simulink model "GPCA_Extension"  (Simulink 7.9)
settings: Solver=ode45  StartTime=0.0  StopTime=inf  RelTol=1e-3
PreLoadFcn:
  | GPCA_Bus_Def
InitFcn:
  | script
values from neighbouring files (symbols this model uses):
  GOutputEvents = [0 0 0 0 0 0 0 0 0 0 0 0 0 0 0 0 0 0 0 0 0]    [script.m]
  GProgrammedDoseRate = 0    [script.m]
  GProgrammedVTBI = 0    [script.m]
libraries: simulink x6
(part 1 of 3)
settings Model: Creator=Yi Zhang  LastModifiedBy=paolo  BufferReuse=off
settings OptimizationCC: OptimizeBlockIOStorage=off  BufferReuse=off  ExpressionFolding=off  LocalBlockOutputs=off  InitFltsAndDblsToZero=on
settings DebuggingCC: FcnCallInpInsideContextMsg=Use local settings  UnconnectedInputMsg=none  UnconnectedOutputMsg=none  BusObjectLabelMismatch=none  StrictBusMsg=Warning
settings SFSimCC: SimParseCustomCode=off
settings GRTTargetCC: CombineOutputUpdateFcns=off  GRTInterface=on

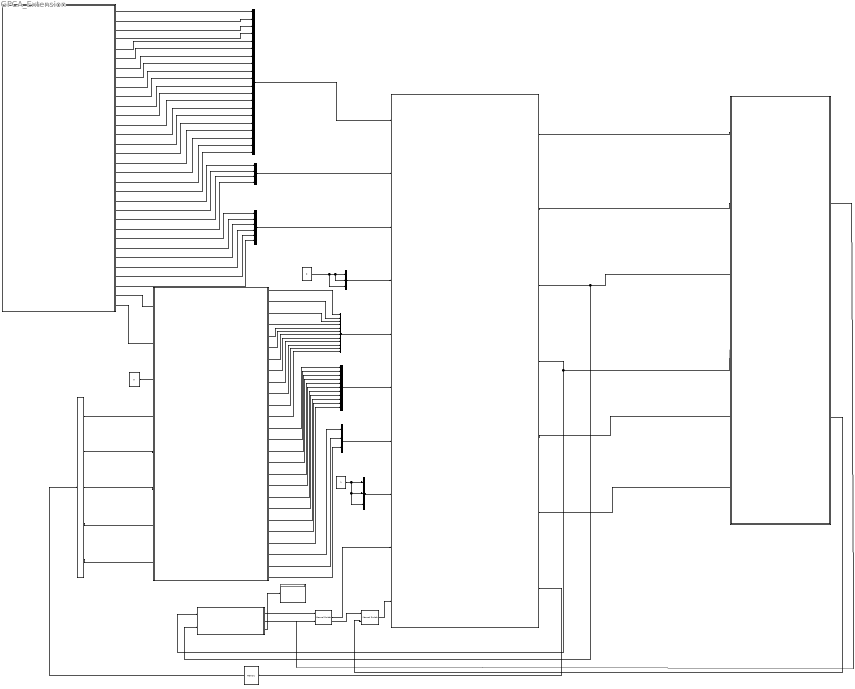
== system GPCA_Extension ==
  note: rrrvr
  1 : Constant  OutDataTypeStr=boolean
  2 : Constant  Value=0  OutDataTypeStr=boolean
  Bus Creator : BusCreator  Tag=DrugLIibraryInput  Description=Readings from the drug library  Inputs=20  OutDataTypeStr=Bus: DrugLibrary
      settings: AttributesFormatString=Drug Library Input
  Bus Creator1 : BusCreator  Description=Readings from the drug library  OutDataTypeStr=Bus: PatientInformation  NonVirtualBus=on
      settings: AttributesFormatString=Patient Information
  Bus Creator2 : BusCreator  Inputs=6  OutDataTypeStr=Bus: DrugInformation  NonVirtualBus=on
      settings: AttributesFormatString=Drug Information
  Bus Creator3 : BusCreator  Inputs=3  OutDataTypeStr=Bus: EnvironmentSensorSignals  NonVirtualBus=on
      settings: AttributesFormatString=Environment Sensor Signals
  Bus Creator4 : BusCreator  Inputs=12  OutDataTypeStr=Bus: HardwareSensorSignals  NonVirtualBus=on
      settings: AttributesFormatString=Hardware Sensor Signals
  Bus Creator5 : BusCreator  Inputs=11  OutDataTypeStr=Bus: InfusionSensorSignals  NonVirtualBus=on
      settings: AttributesFormatString=Infusion Sensor Signals
  Bus Creator7 : BusCreator  Inputs=3  OutDataTypeStr=Bus: InfusionStatus  NonVirtualBus=on
      settings: AttributesFormatString=Infusion Status
  Bus Creator8 : BusCreator  Inputs=3  OutDataTypeStr=Bus: PumpConfigurationsStatus  NonVirtualBus=on
      settings: AttributesFormatString=Pump Configuration Status
  Bus Selector : BusSelector  OutputSignals=signal1,signal3,signal2,O_ProgrammedFlowRate,O_ProgrammedVTBI
  Constant5 : Constant  Value=0
  Display GPCA-UI Port : Display
  Drug/Drug Library/Patient Information Reader : Subsystem
  GPCA Software Controller : Subsystem
  M2 : Memory  InheritSampleTime=on
  Manual Switch Infusion Parameters : simulink/Signal Routing/Manual Switch  sw=1  action=0  varsize=off
  Manual Switch User Actions : simulink/Signal Routing/Manual Switch  sw=1  action=0  varsize=off
  Pump Controller Subsystem : Subsystem
  UI : Subsystem
  WebSocketsBridge : Subsystem
  wires:
  Bus Creator/1 -> GPCA Software Controller/1(Drug Library Input)
  Bus Creator1/1 -> GPCA Software Controller/2(Patient Information Input)
  Bus Creator3/1 -> GPCA Software Controller/4(Environment Sensor Signals)
  Bus Creator4/1 -> GPCA Software Controller/5(Hardware Sensor Signals)
  Bus Creator7/1 -> GPCA Software Controller/7(Infusion Status Input)
  GPCA Software Controller/1(Drug Library Output) -> UI/1(Drug Lib)
  GPCA Software Controller/2(Patient Information Output) -> UI/2(Patient Info)
  GPCA Software Controller/4(Current State) -> WebSocketsBridge/1(CurrentState), UI/4(Current State)
  GPCA Software Controller/6(Alarming Condition) -> UI/6(Alarming Cond)
  GPCA Software Controller/3(Infusion Status Output) -> UI/3(Infusion Status), WebSocketsBridge/2(Infusion Status)
  GPCA Software Controller/5(Drug Information Output) -> UI/5(Drug Info)
  1/1 -> Bus Creator8/1, Bus Creator8/2, Bus Creator8/3
  Bus Creator8/1 -> GPCA Software Controller/8(Pump Configuration Status Input)
  Bus Creator5/1 -> GPCA Software Controller/6(Infusion Sensor Signals)
  GPCA Software Controller/7(Infusion Instructions Output) -> M2/1
  Bus Selector/3 -> Pump Controller Subsystem/6(Infusion Paused)  "<signal2>"
  Bus Selector/2 -> Pump Controller Subsystem/5(Bolus Requested)  "<signal3>"
  Bus Selector/5 -> Pump Controller Subsystem/8(Programmed VTBI)  "<O_ProgrammedVTBI>"
  Bus Selector/1 -> Pump Controller Subsystem/4(Infusion In Progress)  "<signal1>"
  Bus Selector/4 -> Pump Controller Subsystem/7(Programmed Flow Rate)  "<O_ProgrammedFlowRate>"
  Constant5/1 -> Pump Controller Subsystem/3(New Bag Inserted)
  Drug/Drug Library/Patient Information Reader/32(Bolus Time) -> Pump Controller Subsystem/2(Bolus Time)
  Drug/Drug Library/Patient Information Reader/31(Bolus Volume) -> Pump Controller Subsystem/1(Bolus Volume)
  Bus Creator2/1 -> GPCA Software Controller/3(Drug Information Input)
  Drug/Drug Library/Patient Information Reader/30(drugVolumeUnit) -> Bus Creator2/6
  Drug/Drug Library/Patient Information Reader/29(drugDoseUnit) -> Bus Creator2/5
  Drug/Drug Library/Patient Information Reader/28(drugConcentration) -> Bus Creator2/4
  Drug/Drug Library/Patient Information Reader/27(drugDiluentVolume) -> Bus Creator2/3
  Drug/Drug Library/Patient Information Reader/26(drugDoseAmount) -> Bus Creator2/2
  Drug/Drug Library/Patient Information Reader/25(drugName) -> Bus Creator2/1
  Drug/Drug Library/Patient Information Reader/24(patientWeight) -> Bus Creator1/4
  Drug/Drug Library/Patient Information Reader/23(patientGender) -> Bus Creator1/3
  Drug/Drug Library/Patient Information Reader/22(patientAge) -> Bus Creator1/2
  Drug/Drug Library/Patient Information Reader/21(patientName) -> Bus Creator1/1
  Drug/Drug Library/Patient Information Reader/20(drugConcentrationLowerSoftLimit) -> Bus Creator/20
  Drug/Drug Library/Patient Information Reader/19(drugConcentrationLowerHardLimit) -> Bus Creator/19
  Drug/Drug Library/Patient Information Reader/18(drugConcentrationUpperSoftLimit) -> Bus Creator/18
  Drug/Drug Library/Patient Information Reader/17(drugConcentrationUpperHardLimit) -> Bus Creator/17
  Drug/Drug Library/Patient Information Reader/16(drugConcentrationTypical) -> Bus Creator/16
  Drug/Drug Library/Patient Information Reader/15(vtbiUnit) -> Bus Creator/15
  Drug/Drug Library/Patient Information Reader/14(vtbiLowerSoftLimit) -> Bus Creator/14
  Drug/Drug Library/Patient Information Reader/1(drugID) -> Bus Creator/1
  Drug/Drug Library/Patient Information Reader/2(amount) -> Bus Creator/2
  Drug/Drug Library/Patient Information Reader/3(diluentVolume) -> Bus Creator/3
  Drug/Drug Library/Patient Information Reader/4(doseRateTypical) -> Bus Creator/4
  Drug/Drug Library/Patient Information Reader/5(doseRateUpperHardLimit) -> Bus Creator/5
  Drug/Drug Library/Patient Information Reader/6(doseRateUpperSoftLimit) -> Bus Creator/6
  Drug/Drug Library/Patient Information Reader/7(doseRateLowerHardLimit) -> Bus Creator/7
  Drug/Drug Library/Patient Information Reader/8(doseRateLowerSoftLimit) -> Bus Creator/8
  Drug/Drug Library/Patient Information Reader/9(doseRateUnit) -> Bus Creator/9
  Drug/Drug Library/Patient Information Reader/10(vtbiTypical) -> Bus Creator/10
  Drug/Drug Library/Patient Information Reader/11(vtbiUpperHardLimit) -> Bus Creator/11
  Drug/Drug Library/Patient Information Reader/12(vtbiUpperSoftLimit) -> Bus Creator/12
  Drug/Drug Library/Patient Information Reader/13(vtbiLowerHardLimit) -> Bus Creator/13
  2/1 -> Bus Creator3/1, Bus Creator3/2, Bus Creator3/3
  Pump Controller Subsystem/1(Log Failure) -> Bus Creator4/1
  Pump Controller Subsystem/2(Watchdog Interrupt) -> Bus Creator4/2
  Pump Controller Subsystem/3(Door Open) -> Bus Creator4/3
  Pump Controller Subsystem/4(Battery Depleted) -> Bus Creator4/4
  Pump Controller Subsystem/5(Battery Low) -> Bus Creator4/5
  Pump Controller Subsystem/6(Battery Charge Error) -> Bus Creator4/6
  Pump Controller Subsystem/7(VoltOutRange) -> Bus Creator4/7
  Pump Controller Subsystem/8(CPU Error) -> Bus Creator4/8
  Pump Controller Subsystem/9(RTCError) -> Bus Creator4/9
  Pump Controller Subsystem/10(MemoryCorrupted) -> Bus Creator4/10
  Pump Controller Subsystem/11(PumpTooHot) -> Bus Creator4/11
  Pump Controller Subsystem/12(PumpOverheat) -> Bus Creator4/12
  Pump Controller Subsystem/13(EmptyReservoir) -> Bus Creator5/1
  Pump Controller Subsystem/14(LowReservoir) -> Bus Creator5/2
  Pump Controller Subsystem/15(Occlusion) -> Bus Creator5/3
  Pump Controller Subsystem/16(RateTooHigh) -> Bus Creator5/4
  Pump Controller Subsystem/17(RateTooLow) -> Bus Creator5/5
  Pump Controller Subsystem/18(LessThanKVO) -> Bus Creator5/6
  Pump Controller Subsystem/19(RateVary) -> Bus Creator5/7
  Pump Controller Subsystem/20(Flow Rate Above Pump Capacity Alarm) -> Bus Creator5/8
  Pump Controller Subsystem/21(PauseLong) -> Bus Creator5/9
  Pump Controller Subsystem/22(PauseTooLong) -> Bus Creator5/10
  Pump Controller Subsystem/23(Air In Line) -> Bus Creator5/11
  Pump Controller Subsystem/24(Bolus In Progress) -> Bus Creator7/1
  Pump Controller Subsystem/25(TotalVolumeInfused) -> Bus Creator7/2
  Pump Controller Subsystem/26(Current Volume) -> Bus Creator7/3
  M2/1 -> Bus Selector/1
  WebSocketsBridge/1(User Actions) -> Manual Switch User Actions/1
  UI/1(User Actions) -> Manual Switch User Actions/2
  Manual Switch User Actions/1 -> GPCA Software Controller/9(User Actions)
  WebSocketsBridge/2(Infusion Parameters) -> Manual Switch Infusion Parameters/1
  Manual Switch Infusion Parameters/1 -> GPCA Software Controller/10(Infusion Parameters Input)
  UI/2(Infusion Parameters) -> Manual Switch Infusion Parameters/2
  WebSocketsBridge/3(Connection Port for the GPCA-UI) -> Display GPCA-UI Port/1

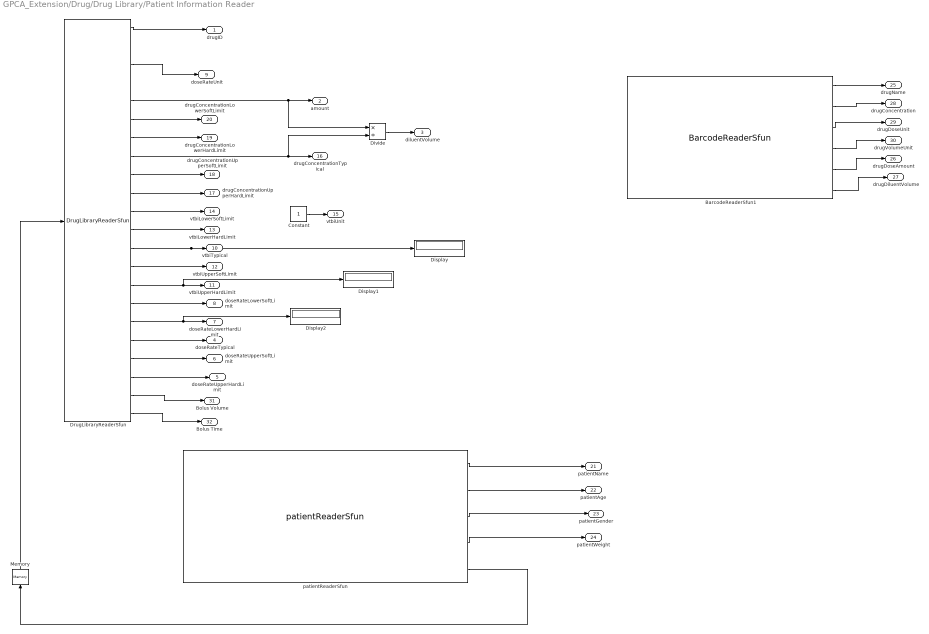
== system GPCA_Extension/Drug/Drug Library/Patient Information Reader ==
  BarcodeReaderSfun1 : S-Function  FunctionName=BarcodeReaderSfun  EnableBusSupport=off  mask(Legacy Function){SFunctionSpec=BarcodeReader(uint32 y1[1], double y2[1], uint32 y3[1], uint32 y4[1], double y5[1], double y6[1]), ShowSpec=on}
      mask prompts: ShowSpec "Display function specification"
      mask help:
      | This block allows you to call the legacy functions specified by the following Legacy Code Tool definition:
      | def.SFunctionName = 'BarcodeReaderSfun';
      | def.OutputFcnSpec = 'BarcodeReader(uint32 y1[1], double y2[1], uint32 y3[1], uint32 y4[1], double y5[1], double y6[1])';
      | def.StartFcnSpec = 'openFile()';
      | def.TerminateFcnSpec = 'closeFile()';
      | def.HeaderFiles = {'BarcodeReaderLCT.h'};
      | def.SourceFiles = {'BarcodeReaderLCT.c'};
      | def.SampleTime = 1;
      mask Help: <p>This block was generated automatically by the Legacy Code Tool. For detailed help on this tool, call<a href="matlab:legacy_code('help')"> legacy_code('help')</a>.</p>
      mask CallbackString:
      | |if strcmp(get_param(gcbh, 'ShowSpec'), 'on')
      |   set_param(gcbh, 'MaskDisplay', sprintf('fprintf(''%s'');', get_param(gcbh, 'SFunctionSpec')));
      | else
      |   set_param(gcbh, 'MaskDisplay', sprintf('fprintf(''%s'');', get_param(gcbh, 'FunctionName')));
      | end
      mask Display: fprintf('BarcodeReader(uint32 y1[1], double y2[1], uint32 y3[1], uint32 y4[1], double y5[1], double y6[1])');
  Constant : Constant  OutDataTypeStr=uint32
  Display : Display
  Display1 : Display
  Display2 : Display
  Divide : Product  Inputs=*/
  DrugLibraryReaderSfun : S-Function  FunctionName=DrugLibraryReaderSfun  EnableBusSupport=off  mask(Legacy Function){SFunctionSpec=DrugLibraryReader(uint32 u1[2], uint32 y1[1], uint32 y2[1], uint32 y3[1], uint32 y4[1], double  y5[1], double  y6[1], double  y7[1],double  y8[1],double  y9[1],double  y10[1],double  y11[1],double  y12[1], double  y13[1],double  y14[1],double  y15[1],double  y16[1],double  y17[1],double  y18[1],double  y19[1], double  y20[1],double  y21[1], uint32  y22[1]), ShowSpec=off}
      mask prompts: ShowSpec "Display function specification"
      mask help:
      | This block allows you to call the legacy functions specified by the following Legacy Code Tool definition:
      | def.SFunctionName = 'DrugLibraryReaderSfun';
      | def.OutputFcnSpec = 'DrugLibraryReader(uint32 u1[2], uint32 y1[1], uint32 y2[1], uint32 y3[1], uint32 y4[1], double  y5[1], double  y6[1], double  y7[1],double  y8[1],double  y9[1],double  y10[1],double  y11[1],double  y12[1], double  y13[1],double  y14[1],double  y15[1],double  y16[1],double  y17[1],double  y18[1],double  y19[1], double  y20[1],double  y21[1], uint32  y22[1])';
      | def.StartFcnSpec = 'openFile()';
      | def.TerminateFcnSpec = 'closeFile()';
      | def.HeaderFiles = {'DrugLibraryLCT.h'};
      | def.SourceFiles = {'DrugLibraryLCT.c'};
      | def.SampleTime = 1;
      mask Help: <p>This block was generated automatically by the Legacy Code Tool. For detailed help on this tool, call<a href="matlab:legacy_code('help')"> legacy_code('help')</a>.</p>
      mask CallbackString:
      | |if strcmp(get_param(gcbh, 'ShowSpec'), 'on')
      |   set_param(gcbh, 'MaskDisplay', sprintf('fprintf(''%s'');', get_param(gcbh, 'SFunctionSpec')));
      | else
      |   set_param(gcbh, 'MaskDisplay', sprintf('fprintf(''%s'');', get_param(gcbh, 'FunctionName')));
      | end
      mask Display: fprintf('DrugLibraryReaderSfun');
  Memory : Memory  InheritSampleTime=on
  patientReaderSfun : S-Function  FunctionName=patientReaderSfun  EnableBusSupport=off  mask(Legacy Function){SFunctionSpec=patientReader(uint32 y1[1], uint32 y2[1], uint32 y3[1], uint32 y4[1], uint32 y5[2]), ShowSpec=on}
      mask prompts: ShowSpec "Display function specification"
      mask help:
      | This block allows you to call the legacy functions specified by the following Legacy Code Tool definition:
      | def.SFunctionName = 'patientReaderSfun';
      | def.InitializeConditionsFcnSpec = 'randomizeSeed()';
      | def.OutputFcnSpec = 'patientReader(uint32 y1[1], uint32 y2[1], uint32 y3[1], uint32 y4[1], uint32 y5[2])';
      | def.StartFcnSpec = 'openFile()';
      | def.TerminateFcnSpec = 'closeFile()';
      | def.HeaderFiles = {'PatientDataReaderLCT.h'};
      | def.SourceFiles = {'PatientDataReaderLCT.c'};
      | def.SampleTime = 1;
      mask Help: <p>This block was generated automatically by the Legacy Code Tool. For detailed help on this tool, call<a href="matlab:legacy_code('help')"> legacy_code('help')</a>.</p>
      mask CallbackString:
      | |if strcmp(get_param(gcbh, 'ShowSpec'), 'on')
      |   set_param(gcbh, 'MaskDisplay', sprintf('fprintf(''%s'');', get_param(gcbh, 'SFunctionSpec')));
      | else
      |   set_param(gcbh, 'MaskDisplay', sprintf('fprintf(''%s'');', get_param(gcbh, 'FunctionName')));
      | end
      mask Display: fprintf('patientReader(uint32 y1[1], uint32 y2[1], uint32 y3[1], uint32 y4[1], uint32 y5[2])');
  drugID : Outport
  amount : Outport  Port=2
  diluentVolume : Outport  Port=3
  doseRateTypical : Outport  Port=4
  doseRateUpperHardLimit : Outport  Port=5
  doseRateUpperSoftLimit : Outport  Port=6
  doseRateLowerHardLimit : Outport  Port=7
  doseRateLowerSoftLimit : Outport  Port=8
  doseRateUnit : Outport  Port=9
  vtbiTypical : Outport  Port=10
  vtbiUpperHardLimit : Outport  Port=11
  vtbiUpperSoftLimit : Outport  Port=12
  vtbiLowerHardLimit : Outport  Port=13
  vtbiLowerSoftLimit : Outport  Port=14
  vtbiUnit : Outport  Port=15
  drugConcentrationTypical : Outport  Port=16
  drugConcentrationUpperHardLimit : Outport  Port=17
  drugConcentrationUpperSoftLimit : Outport  Port=18
  drugConcentrationLowerHardLimit : Outport  Port=19
  drugConcentrationLowerSoftLimit : Outport  Port=20
  patientName : Outport  Port=21
  patientAge : Outport  Port=22
  patientGender : Outport  Port=23
  patientWeight : Outport  Port=24
  drugName : Outport  Port=25
  drugDoseAmount : Outport  Port=26
  drugDiluentVolume : Outport  Port=27
  drugConcentration : Outport  Port=28
  drugDoseUnit : Outport  Port=29
  drugVolumeUnit : Outport  Port=30
  Bolus Volume : Outport  Port=31
  Bolus Time : Outport  Port=32
  wires:
  patientReaderSfun/5 -> Memory/1
  Memory/1 -> DrugLibraryReaderSfun/1
  Divide/1 -> diluentVolume/1
  Constant/1 -> vtbiUnit/1
  patientReaderSfun/1 -> patientName/1
  patientReaderSfun/2 -> patientAge/1
  patientReaderSfun/3 -> patientGender/1
  patientReaderSfun/4 -> patientWeight/1
  BarcodeReaderSfun1/1 -> drugName/1
  BarcodeReaderSfun1/2 -> drugConcentration/1
  BarcodeReaderSfun1/3 -> drugDoseUnit/1
  BarcodeReaderSfun1/4 -> drugVolumeUnit/1
  BarcodeReaderSfun1/5 -> drugDoseAmount/1
  BarcodeReaderSfun1/6 -> drugDiluentVolume/1
  DrugLibraryReaderSfun/1 -> drugID/1
  DrugLibraryReaderSfun/5 -> amount/1, Divide/1
  DrugLibraryReaderSfun/6 -> drugConcentrationLowerSoftLimit/1
  DrugLibraryReaderSfun/7 -> drugConcentrationLowerHardLimit/1
  DrugLibraryReaderSfun/8 -> drugConcentrationTypical/1, Divide/2
  DrugLibraryReaderSfun/9 -> drugConcentrationUpperSoftLimit/1
  DrugLibraryReaderSfun/10 -> drugConcentrationUpperHardLimit/1
  DrugLibraryReaderSfun/11 -> vtbiLowerSoftLimit/1
  DrugLibraryReaderSfun/12 -> vtbiLowerHardLimit/1
  DrugLibraryReaderSfun/13 -> vtbiTypical/1, Display/1
  DrugLibraryReaderSfun/14 -> vtbiUpperSoftLimit/1
  DrugLibraryReaderSfun/15 -> vtbiUpperHardLimit/1, Display1/1
  DrugLibraryReaderSfun/16 -> doseRateLowerSoftLimit/1
  DrugLibraryReaderSfun/17 -> doseRateLowerHardLimit/1, Display2/1
  DrugLibraryReaderSfun/18 -> doseRateTypical/1
  DrugLibraryReaderSfun/19 -> doseRateUpperSoftLimit/1
  DrugLibraryReaderSfun/20 -> doseRateUpperHardLimit/1
  DrugLibraryReaderSfun/3 -> doseRateUnit/1
  DrugLibraryReaderSfun/21 -> Bolus Volume/1
  DrugLibraryReaderSfun/22 -> Bolus Time/1

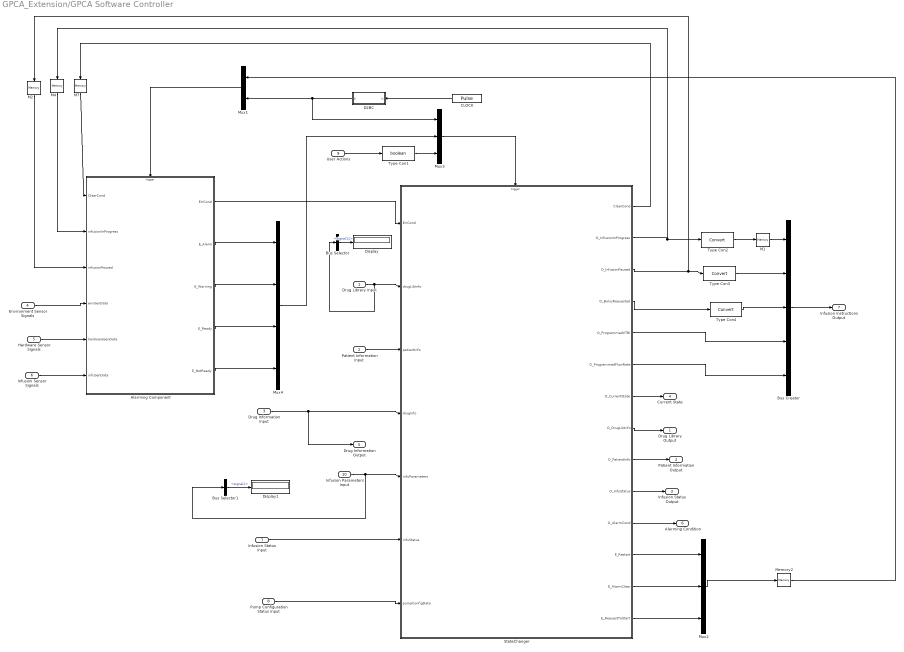
== system GPCA_Extension/GPCA Software Controller ==
  Drug Library Input : Inport
  Patient Information Input : Inport  Port=2
  Drug Information Input : Inport  Port=3
  Environment Sensor Signals : Inport  Port=4
  Hardware Sensor Signals : Inport  Port=5
  Infusion Sensor Signals : Inport  Port=6
  Infusion Status Input : Inport  Port=7
  Pump Configuration Status Input : Inport  Port=8
  User Actions : Inport  Port=9
  Infusion Parameters Input : Inport  Port=10
  Alarming Component : Stateflow chart  TreatAsAtomicUnit=on
  Bus Creator : BusCreator  Inputs=5  OutDataTypeStr=Bus: InfusionInstructions  NonVirtualBus=on
  Bus Selector : BusSelector  OutputSignals=signal11
  Bus Selector1 : BusSelector  OutputSignals=signal1
  CLOCK : DiscretePulseGenerator  PulseType=Time based  PulseWidth=50
  D2BC : MATLAB Function  TreatAsAtomicUnit=on
  Display : Display
  Display1 : Display
  M{1..2,4,7} (4 alike) : Memory  InheritSampleTime=on
  Memory2 : Memory  InheritSampleTime=on
  Mux1 : Mux  Inputs=2
  Mux2 : Mux  Inputs=3
  Mux3 : Mux  Inputs=3
  Mux4 : Mux
  StateChanger : Stateflow chart  TreatAsAtomicUnit=on
  Type Con1 : DataTypeConversion  OutDataTypeStr=boolean
  Type Con2 : DataTypeConversion
  Type Con3 : DataTypeConversion
  Type Con4 : DataTypeConversion
  Drug Library Output : Outport
  Patient Information Output : Outport  Port=2
  Infusion Status Output : Outport  Port=3
  Current State : Outport  Port=4
  Drug Information Output : Outport  Port=5
  Alarming Condition : Outport  Port=6
  Infusion Instructions Output : Outport  Port=7
  wires:
  StateChanger/1(ClearCond) -> M7/1
  Mux3/1 -> StateChanger/Trigger
  Mux1/1 -> Alarming Component/Trigger
  StateChanger/2(O_InfusionInProgress) -> M4/1, Type Con2/1
  Alarming Component/1(ErrCond) -> StateChanger/1(ErrCond)
  StateChanger/12(E_Restart) -> Mux2/1
  StateChanger/13(E_AlarmClear) -> Mux2/2
  StateChanger/14(E_RequestToStart) -> Mux2/3
  Mux2/1 -> Memory2/1
  CLOCK/1 -> D2BC/1(u)
  D2BC/1(y) -> Mux1/2, Mux3/1
  Alarming Component/2(E_Alarm) -> Mux4/1
  Alarming Component/3(E_Warning) -> Mux4/2
  Alarming Component/4(E_Ready) -> Mux4/3
  Alarming Component/5(E_NotReady) -> Mux4/4
  Mux4/1 -> Mux3/2
  Type Con2/1 -> M1/1
  Memory2/1 -> Mux1/1
  Environment Sensor Signals/1 -> Alarming Component/4(envSenData)
  Hardware Sensor Signals/1 -> Alarming Component/5(hardwareSenData)
  Infusion Sensor Signals/1 -> Alarming Component/6(infuSenData)
  Drug Library Input/1 -> StateChanger/2(drugLibInfo), Bus Selector/1
  Patient Information Input/1 -> StateChanger/3(patientInfo)
  Drug Information Input/1 -> StateChanger/4(drugInfo), Drug Information Output/1
  Infusion Parameters Input/1 -> StateChanger/5(infuParameters), Bus Selector1/1
  Infusion Status Input/1 -> StateChanger/6(infuStatus)
  Pump Configuration Status Input/1 -> StateChanger/7(pumpConfigData)
  StateChanger/11(O_AlarmCond) -> Alarming Condition/1
  StateChanger/7(O_CurrentState) -> Current State/1
  StateChanger/9(O_PatientInfo) -> Patient Information Output/1
  StateChanger/8(O_DrugLibInfo) -> Drug Library Output/1
  M1/1 -> Bus Creator/1
  StateChanger/3(O_InfusionPaused) -> M2/1, Type Con3/1
  Bus Creator/1 -> Infusion Instructions Output/1
  M7/1 -> Alarming Component/1(ClearCond)
  M4/1 -> Alarming Component/2(infusionInProgress)
  M2/1 -> Alarming Component/3(infusionPaused)
  StateChanger/4(O_BolusRequested) -> Type Con4/1
  StateChanger/5(O_ProgrammedVTBI) -> Bus Creator/4
  StateChanger/6(O_ProgrammedFlowRate) -> Bus Creator/5
  Type Con3/1 -> Bus Creator/2
  Type Con4/1 -> Bus Creator/3
  StateChanger/10(O_InfuStatus) -> Infusion Status Output/1
  Type Con1/1 -> Mux3/3
  User Actions/1 -> Type Con1/1
  Bus Selector/1 -> Display/1  "<signal11>"
  Bus Selector1/1 -> Display1/1  "<signal1>"

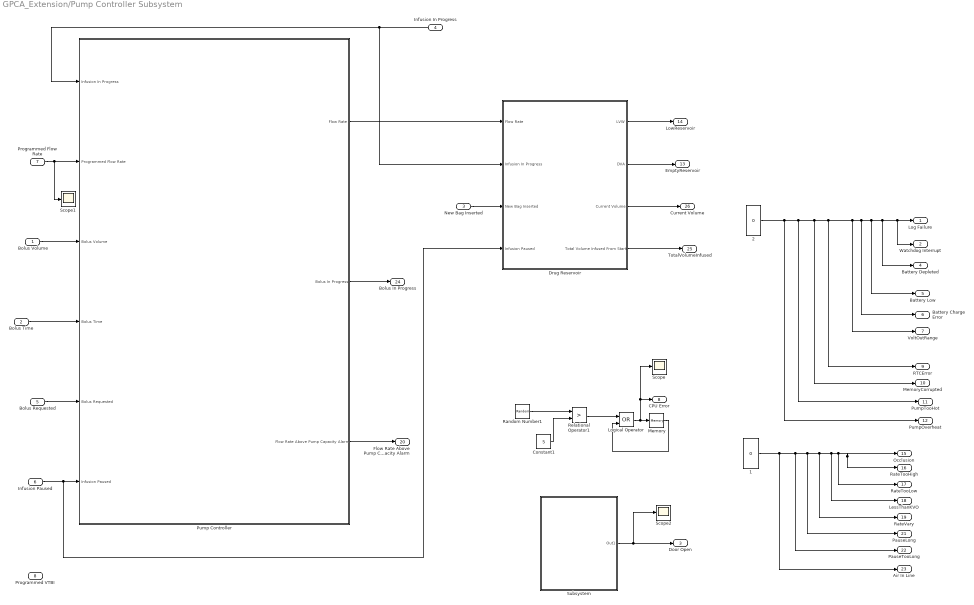
== system GPCA_Extension/Pump Controller Subsystem ==
  Bolus Volume : Inport
  Bolus Time : Inport  Port=2
  New Bag Inserted : Inport  Port=3
  Infusion In Progress : Inport  Port=4
  Bolus Requested : Inport  Port=5
  Infusion Paused : Inport  Port=6
  Programmed Flow Rate : Inport  Port=7
  Programmed VTBI : Inport  Port=8
  1 : Constant  Value=0  OutDataTypeStr=boolean
  2 : Constant  Value=0  OutDataTypeStr=boolean
  Constant1 : Constant  Value=5
  Drug Reservoir : Subsystem
  Logical Operator : Logic  Operator=OR  AllPortsSameDT=off  OutDataTypeStr=boolean
  Memory : Memory
  Pump Controller : Subsystem
  Random Number1 : RandomNumber  Mean=0.5
  Relational Operator1 : RelationalOperator  Operator=>  OutDataTypeStr=boolean
  Scope : Scope
      settings: YMin=1  YMax=1
  Scope1 : Scope
      settings: YMin=1.25  YMax=1.25
  Scope2 : Scope
      settings: YMin=-1  YMax=1  SaveName=ScopeData2
  Subsystem : Subsystem
  Log Failure : Outport
  Watchdog Interrupt : Outport  Port=2
  Door Open : Outport  Port=3
  Battery Depleted : Outport  Port=4
  Battery Low : Outport  Port=5
  Battery Charge Error : Outport  Port=6
  VoltOutRange : Outport  Port=7
  CPU Error : Outport  Port=8
  RTCError : Outport  Port=9
  MemoryCorrupted : Outport  Port=10
  PumpTooHot : Outport  Port=11
  PumpOverheat : Outport  Port=12
  EmptyReservoir : Outport  Port=13
  LowReservoir : Outport  Port=14
  Occlusion : Outport  Port=15
  RateTooHigh : Outport  Port=16
  RateTooLow : Outport  Port=17
  LessThanKVO : Outport  Port=18
  RateVary : Outport  Port=19
  Flow Rate Above Pump Capacity Alarm : Outport  Port=20
  PauseLong : Outport  Port=21
  PauseTooLong : Outport  Port=22
  Air In Line : Outport  Port=23
  Bolus In Progress : Outport  Port=24
  TotalVolumeInfused : Outport  Port=25
  Current Volume : Outport  Port=26
  wires:
  Bolus Requested/1 -> Pump Controller/5(Bolus Requested)
  Pump Controller/2(Bolus In Progress) -> Bolus In Progress/1
  Infusion Paused/1 -> Pump Controller/6(Infusion Paused), Drug Reservoir/4(Infusion Paused)
  New Bag Inserted/1 -> Drug Reservoir/3(New Bag Inserted)
  Drug Reservoir/3(Current Volume) -> Current Volume/1
  Drug Reservoir/2(DVA) -> EmptyReservoir/1
  Drug Reservoir/4(Total Volume Infused From Start) -> TotalVolumeInfused/1
  Infusion In Progress/1 -> Pump Controller/1(Infusion In Progress), Drug Reservoir/2(Infusion In Progress)
  Programmed Flow Rate/1 -> Pump Controller/2(Programmed Flow Rate), Scope1/1
  Drug Reservoir/1(LVW) -> LowReservoir/1
  Pump Controller/3(Flow Rate Above Pump Capacity Alarm) -> Flow Rate Above Pump Capacity Alarm/1
  Bolus Time/1 -> Pump Controller/4(Bolus Time)
  Bolus Volume/1 -> Pump Controller/3(Bolus Volume)
  2/1 -> RTCError/1, Battery Charge Error/1, Battery Low/1, Log Failure/1, Watchdog Interrupt/1, Battery Depleted/1, VoltOutRange/1, MemoryCorrupted/1, PumpTooHot/1, PumpOverheat/1
  1/1 -> RateTooLow/1, RateTooHigh/1, Occlusion/1, LessThanKVO/1, RateVary/1, PauseLong/1, PauseTooLong/1, Air In Line/1
  Pump Controller/1(Flow Rate) -> Drug Reservoir/1(Flow Rate)
  Random Number1/1 -> Relational Operator1/1
  Constant1/1 -> Relational Operator1/2
  Relational Operator1/1 -> Logical Operator/1
  Logical Operator/1 -> Memory/1, CPU Error/1, Scope/1
  Memory/1 -> Logical Operator/2
  Subsystem/1(Out1) -> Scope2/1, Door Open/1

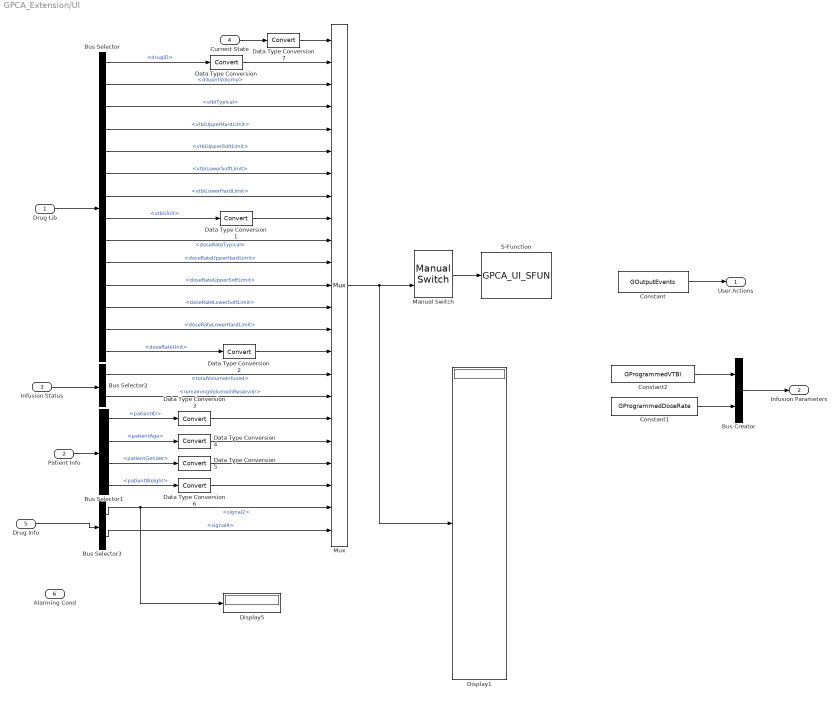
== system GPCA_Extension/UI ==
  Drug Lib : Inport
  Patient Info : Inport  Port=2
  Infusion Status : Inport  Port=3
  Current State : Inport  Port=4
  Drug Info : Inport  Port=5
  Alarming Cond : Inport  Port=6
  Bus Creator : BusCreator  Inputs=2  OutDataTypeStr=Bus: InfusionParameters
  Bus Selector : BusSelector  OutputSignals=drugID,diluentVolume,vtbiTypical,vtbiUpperHardLimit,vtbiUpperSoftLimit,vtbiLowerSoftLimit,vtbiLowerHardLimit,vtbiUnit,doseRateTypical,doseRateUpperHardLimit,doseRateUpperSoftLimit,doseRateLowerSoftLimit,doseRateLowerHardLimit,doseRateUnit
  Bus Selector1 : BusSelector  OutputSignals=patientID,patientAge,patientGender,patientWeight
  Bus Selector2 : BusSelector  OutputSignals=totalVolumeInfused,remainingVolumeInReservoir
  Bus Selector3 : BusSelector  OutputSignals=signal2,signal4
  Constant : Constant  Value=GOutputEvents
  Constant1 : Constant  Value=GProgrammedDoseRate
  Constant2 : Constant  Value=GProgrammedVTBI
  Data Type Conversion{,1..7} (8 alike) : DataTypeConversion
  Display1 : Display
  Display5 : Display
  Manual Switch : simulink/Signal Routing/Manual Switch  sw=0  action=0  varsize=off
  Mux : Mux  Inputs=23
  S-Function : S-Function  FunctionName=GPCA_UI_SFUN  EnableBusSupport=off
  User Actions : Outport
  Infusion Parameters : Outport  Port=2
  wires:
  Current State/1 -> Data Type Conversion7/1
  Drug Lib/1 -> Bus Selector/1
  Bus Selector/1 -> Data Type Conversion/1  "<drugID>"
  Bus Selector/2 -> Mux/3  "<diluentVolume>"
  Bus Selector/3 -> Mux/4  "<vtbiTypical>"
  Bus Selector/4 -> Mux/5  "<vtbiUpperHardLimit>"
  Bus Selector/5 -> Mux/6  "<vtbiUpperSoftLimit>"
  Bus Selector/6 -> Mux/7  "<vtbiLowerSoftLimit>"
  Bus Selector/7 -> Mux/8  "<vtbiLowerHardLimit>"
  Bus Selector/8 -> Data Type Conversion1/1  "<vtbiUnit>"
  Bus Selector/9 -> Mux/10  "<doseRateTypical>"
  Bus Selector/10 -> Mux/11  "<doseRateUpperHardLimit>"
  Bus Selector/11 -> Mux/12  "<doseRateUpperSoftLimit>"
  Bus Selector/12 -> Mux/13  "<doseRateLowerSoftLimit>"
  Bus Selector/13 -> Mux/14  "<doseRateLowerHardLimit>"
  Bus Selector/14 -> Data Type Conversion2/1  "<doseRateUnit>"
  Patient Info/1 -> Bus Selector1/1
  Bus Selector1/1 -> Data Type Conversion3/1  "<patientID>"
  Bus Selector1/2 -> Data Type Conversion4/1  "<patientAge>"
  Bus Selector1/3 -> Data Type Conversion5/1  "<patientGender>"
  Bus Selector1/4 -> Data Type Conversion6/1  "<patientWeight>"
  Bus Selector3/1 -> Mux/22, Display5/1  "<signal2>"
  Bus Selector3/2 -> Mux/23  "<signal4>"
  Data Type Conversion/1 -> Mux/2
  Data Type Conversion1/1 -> Mux/9
  Data Type Conversion2/1 -> Mux/15
  Data Type Conversion3/1 -> Mux/18
  Data Type Conversion4/1 -> Mux/19
  Data Type Conversion5/1 -> Mux/20
  Data Type Conversion6/1 -> Mux/21
  Infusion Status/1 -> Bus Selector2/1
  Drug Info/1 -> Bus Selector3/1
  Constant/1 -> User Actions/1
  Constant2/1 -> Bus Creator/1
  Constant1/1 -> Bus Creator/2
  Bus Creator/1 -> Infusion Parameters/1
  Bus Selector2/1 -> Mux/16  "<totalVolumeInfused>"
  Bus Selector2/2 -> Mux/17  "<remainingVolumeInReservoir>"
  Data Type Conversion7/1 -> Mux/1
  Mux/1 -> Display1/1, Manual Switch/2
  Manual Switch/1 -> S-Function/1

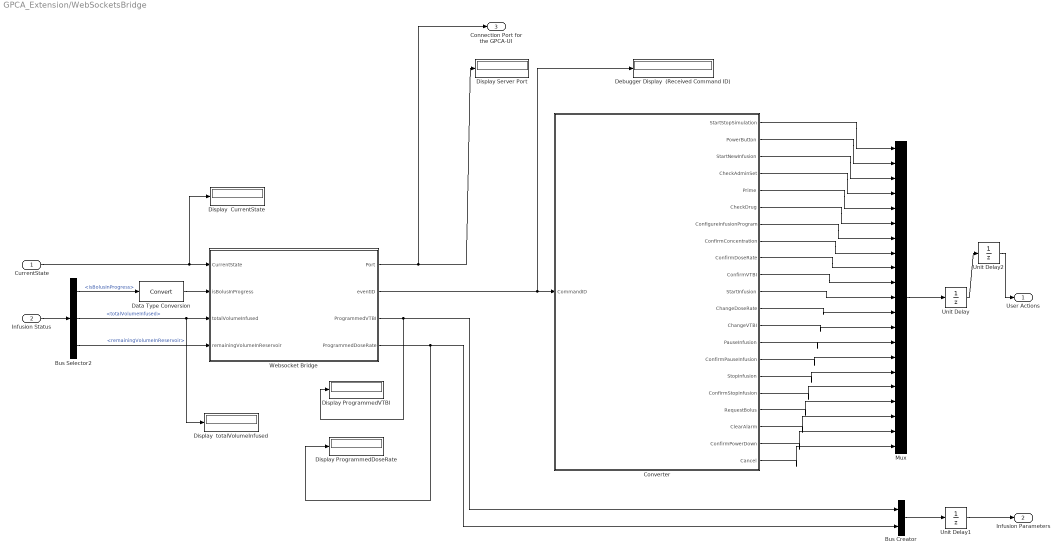
== system GPCA_Extension/WebSocketsBridge ==
  CurrentState : Inport
  Infusion Status : Inport  Port=2
  Bus Creator : BusCreator  Inputs=2  OutDataTypeStr=Bus: InfusionParameters
  Bus Selector2 : BusSelector  OutputSignals=isBolusInProgress,totalVolumeInfused,remainingVolumeInReservoir
  Converter : Stateflow chart  TreatAsAtomicUnit=on
  Data Type Conversion : DataTypeConversion
  Debugger Display  (Received Command ID) : Display
  Display ProgrammedDoseRate : Display
  Display ProgrammedVTBI : Display
  Display Server Port : Display
  Display  CurrentState : Display
  Display  totalVolumeInfused : Display
  Mux : Mux  Inputs=21
  Unit Delay : UnitDelay  SampleTime=-1
  Unit Delay1 : UnitDelay  SampleTime=-1
  Unit Delay2 : UnitDelay  SampleTime=-1
  Websocket Bridge : Subsystem
  User Actions : Outport
  Infusion Parameters : Outport  Port=2
  Connection Port for the GPCA-UI : Outport  Port=3
  wires:
  Converter/1(StartStopSimulation) -> Mux/1
  Converter/2(PowerButton) -> Mux/2
  Converter/3(StartNewInfusion) -> Mux/3
  Converter/4(CheckAdminSet) -> Mux/4
  Converter/5(Prime) -> Mux/5
  Converter/6(CheckDrug) -> Mux/6
  Converter/7(ConfigureInfusionProgram) -> Mux/7
  Converter/8(ConfirmConcentration) -> Mux/8
  Converter/9(ConfirmDoseRate) -> Mux/9
  Converter/10(ConfirmVTBI) -> Mux/10
  Converter/11(StartInfusion) -> Mux/11
  Converter/12(ChangeDoseRate) -> Mux/12
  Converter/13(ChangeVTBI) -> Mux/13
  Converter/14(PauseInfusion) -> Mux/14
  Converter/15(ConfirmPauseInfusion) -> Mux/15
  Converter/16(StopInfusion) -> Mux/16
  Converter/17(ConfirmStopInfusion) -> Mux/17
  Converter/18(RequestBolus) -> Mux/18
  Converter/19(ClearAlarm) -> Mux/19
  Converter/20(ConfirmPowerDown) -> Mux/20
  Converter/21(Cancel) -> Mux/21
  Websocket Bridge/2(eventID) -> Debugger Display  (Received Command ID)/1, Converter/1(CommandID)
  Websocket Bridge/1(Port) -> Display Server Port/1, Connection Port for the GPCA-UI/1
  Websocket Bridge/3(ProgrammedVTBI) -> Bus Creator/1, Display ProgrammedVTBI/1
  Websocket Bridge/4(ProgrammedDoseRate) -> Bus Creator/2, Display ProgrammedDoseRate/1
  CurrentState/1 -> Websocket Bridge/1(CurrentState), Display  CurrentState/1
  Mux/1 -> Unit Delay/1
  Bus Selector2/3 -> Websocket Bridge/4(remainingVolumeInReservoir)  "<remainingVolumeInReservoir>"
  Bus Selector2/2 -> Websocket Bridge/3(totalVolumeInfused), Display  totalVolumeInfused/1  "<totalVolumeInfused>"
  Infusion Status/1 -> Bus Selector2/1
  Bus Selector2/1 -> Data Type Conversion/1  "<isBolusInProgress>"
  Data Type Conversion/1 -> Websocket Bridge/2(isBolusInProgress)
  Bus Creator/1 -> Unit Delay1/1
  Unit Delay1/1 -> Infusion Parameters/1
  Unit Delay/1 -> Unit Delay2/1
  Unit Delay2/1 -> User Actions/1

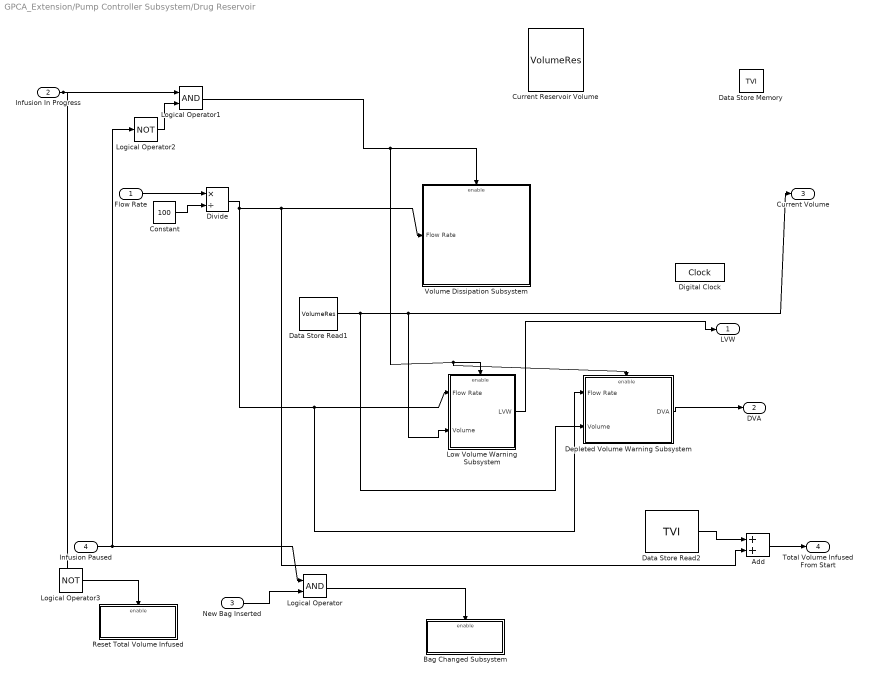
== system GPCA_Extension/Pump Controller Subsystem/Drug Reservoir ==
  Flow Rate : Inport
  Infusion In Progress : Inport  Port=2
  New Bag Inserted : Inport  Port=3
  Infusion Paused : Inport  Port=4
  Add : Sum
  Bag Changed Subsystem : Subsystem  TreatAsAtomicUnit=on
  Constant : Constant  Value=100
  Current Reservoir Volume : DataStoreMemory  DataStoreName=VolumeRes  InitialValue=2500
  Data Store Memory : DataStoreMemory  DataStoreName=TVI
  Data Store Read1 : DataStoreRead  DataStoreName=VolumeRes
      settings: AttributesFormatString=1
  Data Store Read2 : DataStoreRead  DataStoreName=TVI
  Depleted Volume Warning Subsystem : Subsystem
  Digital Clock : DigitalClock
  Divide : Product  Inputs=*/
  Logical Operator : Logic  AllPortsSameDT=off  OutDataTypeStr=boolean
  Logical Operator1 : Logic  AllPortsSameDT=off  OutDataTypeStr=boolean
  Logical Operator2 : Logic  Operator=NOT  AllPortsSameDT=off  OutDataTypeStr=boolean
  Logical Operator3 : Logic  Operator=NOT  AllPortsSameDT=off  OutDataTypeStr=boolean
  Low Volume Warning Subsystem : Subsystem
  Reset Total Volume Infused : Subsystem  TreatAsAtomicUnit=on
  Volume Dissipation Subsystem : Subsystem
  LVW : Outport
  DVA : Outport  Port=2
  Current Volume : Outport  Port=3
  Total Volume Infused From Start : Outport  Port=4
  wires:
  Divide/1 -> Low Volume Warning Subsystem/1(Flow Rate), Depleted Volume Warning Subsystem/1(Flow Rate), Volume Dissipation Subsystem/1(Flow Rate), Add/2
  Logical Operator1/1 -> Volume Dissipation Subsystem/Enable, Low Volume Warning Subsystem/Enable, Depleted Volume Warning Subsystem/Enable
  Depleted Volume Warning Subsystem/1(DVA) -> DVA/1
  Low Volume Warning Subsystem/1(LVW) -> LVW/1
  Data Store Read1/1 -> Depleted Volume Warning Subsystem/2(Volume), Low Volume Warning Subsystem/2(Volume), Current Volume/1
  Infusion Paused/1 -> Logical Operator/1, Logical Operator2/1
  New Bag Inserted/1 -> Logical Operator/2
  Logical Operator/1 -> Bag Changed Subsystem/Enable
  Data Store Read2/1 -> Add/1
  Add/1 -> Total Volume Infused From Start/1
  Flow Rate/1 -> Divide/1
  Constant/1 -> Divide/2
  Infusion In Progress/1 -> Logical Operator1/1, Logical Operator3/1
  Logical Operator2/1 -> Logical Operator1/2
  Logical Operator3/1 -> Reset Total Volume Infused/Enable

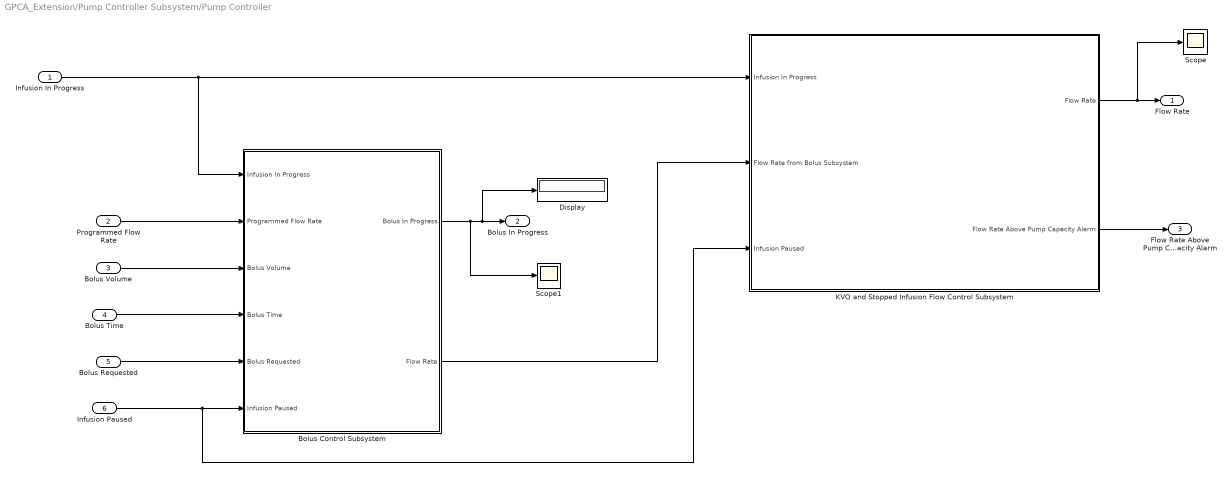
== system GPCA_Extension/Pump Controller Subsystem/Pump Controller ==
  Infusion In Progress : Inport
  Programmed Flow Rate : Inport  Port=2
  Bolus Volume : Inport  Port=3
  Bolus Time : Inport  Port=4
  Bolus Requested : Inport  Port=5
  Infusion Paused : Inport  Port=6
  Bolus Control Subsystem : Subsystem
  Display : Display
  KVO and Stopped Infusion Flow Control Subsystem : Subsystem
  Scope : Scope
      settings: YMin=1.25  YMax=1.25  SaveName=ScopeData3
  Scope1 : Scope
      settings: YMin=-1  YMax=1  SaveName=ScopeData4
  Flow Rate : Outport
  Bolus In Progress : Outport  Port=2
  Flow Rate Above Pump Capacity Alarm : Outport  Port=3
  wires:
  Infusion In Progress/1 -> KVO and Stopped Infusion Flow Control Subsystem/1(Infusion In Progress), Bolus Control Subsystem/1(Infusion In Progress)
  Programmed Flow Rate/1 -> Bolus Control Subsystem/2(Programmed Flow Rate)
  Bolus Requested/1 -> Bolus Control Subsystem/5(Bolus Requested)
  Bolus Volume/1 -> Bolus Control Subsystem/3(Bolus Volume)
  Bolus Time/1 -> Bolus Control Subsystem/4(Bolus Time)
  Bolus Control Subsystem/1(" Bolus In Progress") -> Scope1/1, Bolus In Progress/1, Display/1
  Infusion Paused/1 -> Bolus Control Subsystem/6(Infusion Paused), KVO and Stopped Infusion Flow Control Subsystem/3(Infusion Paused)
  Bolus Control Subsystem/2(Flow Rate) -> KVO and Stopped Infusion Flow Control Subsystem/2(Flow Rate from Bolus Subsystem)
  KVO and Stopped Infusion Flow Control Subsystem/1(Flow Rate) -> Flow Rate/1, Scope/1
  KVO and Stopped Infusion Flow Control Subsystem/2(" Flow Rate Above Pump Capacity Alarm") -> Flow Rate Above Pump Capacity Alarm/1

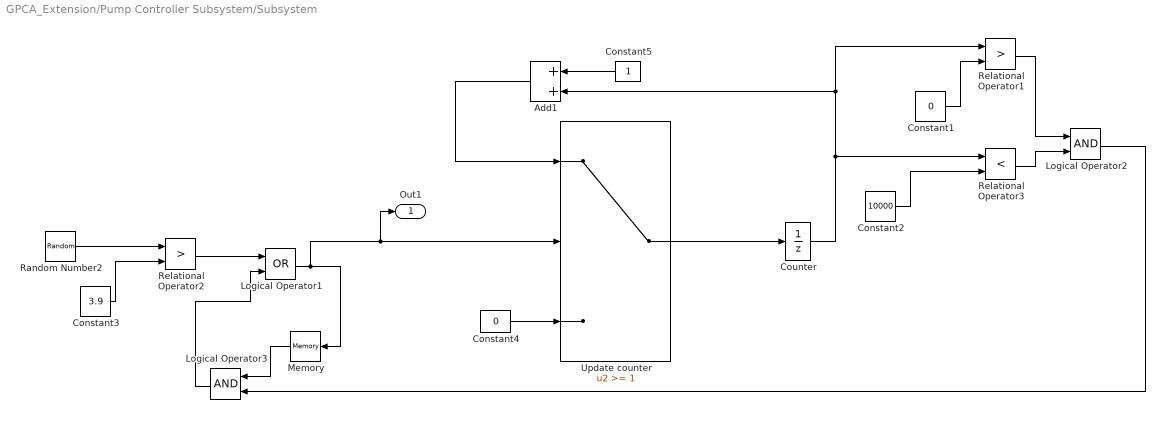
== system GPCA_Extension/Pump Controller Subsystem/Subsystem ==
  Add1 : Sum
  Constant1 : Constant  Value=0
  Constant2 : Constant  Value=10000
  Constant3 : Constant  Value=3.9
  Constant4 : Constant  Value=0
  Constant5 : Constant
  Counter : UnitDelay
  Logical Operator1 : Logic  Operator=OR  AllPortsSameDT=off  OutDataTypeStr=boolean
  Logical Operator2 : Logic  AllPortsSameDT=off  OutDataTypeStr=boolean
  Logical Operator3 : Logic  AllPortsSameDT=off  OutDataTypeStr=boolean
  Memory : Memory
  Random Number2 : RandomNumber  Mean=0.5
  Relational Operator1 : RelationalOperator  Operator=>  OutDataTypeStr=boolean
  Relational Operator2 : RelationalOperator  Operator=>  OutDataTypeStr=boolean
  Relational Operator3 : RelationalOperator  Operator=<  OutDataTypeStr=boolean
  Update counter : Switch  Threshold=1
  Out1 : Outport
  wires:
  Random Number2/1 -> Relational Operator2/1
  Constant3/1 -> Relational Operator2/2
  Relational Operator2/1 -> Logical Operator1/1
  Logical Operator1/1 -> Memory/1, Update counter/2, Out1/1
  Add1/1 -> Update counter/1
  Constant5/1 -> Add1/1
  Counter/1 -> Relational Operator3/1, Add1/2, Relational Operator1/1
  Update counter/1 -> Counter/1
  Constant4/1 -> Update counter/3
  Constant2/1 -> Relational Operator3/2
  Relational Operator3/1 -> Logical Operator2/2
  Constant1/1 -> Relational Operator1/2
  Relational Operator1/1 -> Logical Operator2/1
  Memory/1 -> Logical Operator3/1
  Logical Operator2/1 -> Logical Operator3/2
  Logical Operator3/1 -> Logical Operator1/2

== system GPCA_Extension/WebSocketsBridge/Websocket Bridge ==
  CurrentState : Inport
  isBolusInProgress : Inport  Port=2
  totalVolumeInfused : Inport  Port=3
  remainingVolumeInReservoir : Inport  Port=4
  tick : DiscretePulseGenerator  PulseType=Time based  Period=512  PulseWidth=50
  websocket_serverLCT : S-Function  FunctionName=websocket_serverLCT  EnableBusSupport=off  mask(Legacy Function){SFunctionSpec=int32 y1 = WebsocketServer(double u1, uint32 u2, uint32 u3, double u4, double u5, uint32 y2[1], double y3[1], double y4[1]), ShowSpec=off}
      mask prompts: ShowSpec "Display function specification"
      mask help:
      | This block allows you to call the legacy functions specified by the following Legacy Code Tool definition:
      | def.SFunctionName = 'websocket_serverLCT';
      | def.OutputFcnSpec = 'int32 y1 = WebsocketServer(double u1, uint32 u2, uint32 u3, double u4, double u5, uint32 y2[1], double y3[1], double y4[1])';
      | def.TerminateFcnSpec = 'close_websocket()';
      | def.HeaderFiles = {'websocket_server.h'};
      | def.SourceFiles = {'websocket_server.c'};
      | def.HostLibFiles = {'libwebsockets.so.0.0.3'};
      mask Help: <p>This block was generated automatically by the Legacy Code Tool. For detailed help on this tool, call<a href="matlab:legacy_code('help')"> legacy_code('help')</a>.</p>
      mask CallbackString:
      | |if strcmp(get_param(gcbh, 'ShowSpec'), 'on')
      |   set_param(gcbh, 'MaskDisplay', sprintf('fprintf(''%s'');', get_param(gcbh, 'SFunctionSpec')));
      | else
      |   set_param(gcbh, 'MaskDisplay', sprintf('fprintf(''%s'');', get_param(gcbh, 'FunctionName')));
      | end
      mask Display: fprintf('websocket_serverLCT');
  Port : Outport
  eventID : Outport  Port=2
  ProgrammedVTBI : Outport  Port=3
  ProgrammedDoseRate : Outport  Port=4
  wires:
  websocket_serverLCT/3 -> ProgrammedVTBI/1
  websocket_serverLCT/4 -> ProgrammedDoseRate/1
  websocket_serverLCT/1 -> Port/1
  websocket_serverLCT/2 -> eventID/1
  CurrentState/1 -> websocket_serverLCT/2
  isBolusInProgress/1 -> websocket_serverLCT/3
  totalVolumeInfused/1 -> websocket_serverLCT/4
  tick/1 -> websocket_serverLCT/1
  remainingVolumeInReservoir/1 -> websocket_serverLCT/5

== system GPCA_Extension/Pump Controller Subsystem/Drug Reservoir/Bag Changed Subsystem ==
  Enable : EnablePort
  Constant : Constant  Value=10
  Data Store Write : DataStoreWrite  DataStoreName=VolumeRes
  wires:
  Constant/1 -> Data Store Write/1

== system GPCA_Extension/Pump Controller Subsystem/Drug Reservoir/Depleted Volume Warning Subsystem ==
  Flow Rate : Inport
  Volume : Inport  Port=2
  Enable : EnablePort
  Compare To Constant : simulink/Logic and Bit Operations/Compare To Constant  relop=<=  const=5  OutDataTypeStr=boolean  ZeroCross=off
  Divide : Product  Inputs=*/
  DVA : Outport
  wires:
  Volume/1 -> Divide/1
  Flow Rate/1 -> Divide/2
  Divide/1 -> Compare To Constant/1
  Compare To Constant/1 -> DVA/1

== system GPCA_Extension/Pump Controller Subsystem/Drug Reservoir/Low Volume Warning Subsystem ==
  Flow Rate : Inport
  Volume : Inport  Port=2
  Enable : EnablePort
  Compare To Constant : simulink/Logic and Bit Operations/Compare To Constant  relop=<=  const=15  OutDataTypeStr=boolean  ZeroCross=off
  Compare To Constant1 : simulink/Logic and Bit Operations/Compare To Constant  relop=>  const=5  OutDataTypeStr=boolean  ZeroCross=off
  Divide : Product  Inputs=*/
  Logical Operator : Logic  AllPortsSameDT=off  OutDataTypeStr=boolean
  LVW : Outport
  wires:
  Volume/1 -> Divide/1
  Flow Rate/1 -> Divide/2
  Divide/1 -> Compare To Constant/1, Compare To Constant1/1
  Compare To Constant1/1 -> Logical Operator/2
  Compare To Constant/1 -> Logical Operator/1
  Logical Operator/1 -> LVW/1

== system GPCA_Extension/Pump Controller Subsystem/Drug Reservoir/Reset Total Volume Infused ==
  Enable : EnablePort
  Constant : Constant  Value=0
  Data Store Write : DataStoreWrite  DataStoreName=TVI
  wires:
  Constant/1 -> Data Store Write/1

== system GPCA_Extension/Pump Controller Subsystem/Drug Reservoir/Volume Dissipation Subsystem ==
  Flow Rate : Inport
  Enable : EnablePort
  Add : Sum
  Data Store Read : DataStoreRead  DataStoreName=VolumeRes
  Data Store Read1 : DataStoreRead  DataStoreName=TVI
  Data Store Write : DataStoreWrite  DataStoreName=VolumeRes
  Data Store Write1 : DataStoreWrite  DataStoreName=TVI
  "Minimum Drug Volume " : Constant  Value=0  OutDataTypeStr=double
  Minimum Drug Volume 1 : Constant  Value=0  OutDataTypeStr=double
  Subtract : Sum  Inputs=+-
  Switch : Switch
  Switch1 : Switch
  wires:
  Data Store Read/1 -> Subtract/1
  Flow Rate/1 -> Subtract/2, Switch/1
  Data Store Read1/1 -> Add/2
  Add/1 -> Data Store Write1/1
  Subtract/1 -> Switch/2, Switch1/1, Switch1/2
  Minimum Drug Volume 1/1 -> Switch/3
  Switch/1 -> Add/1
  "Minimum Drug Volume "/1 -> Switch1/3
  Switch1/1 -> Data Store Write/1

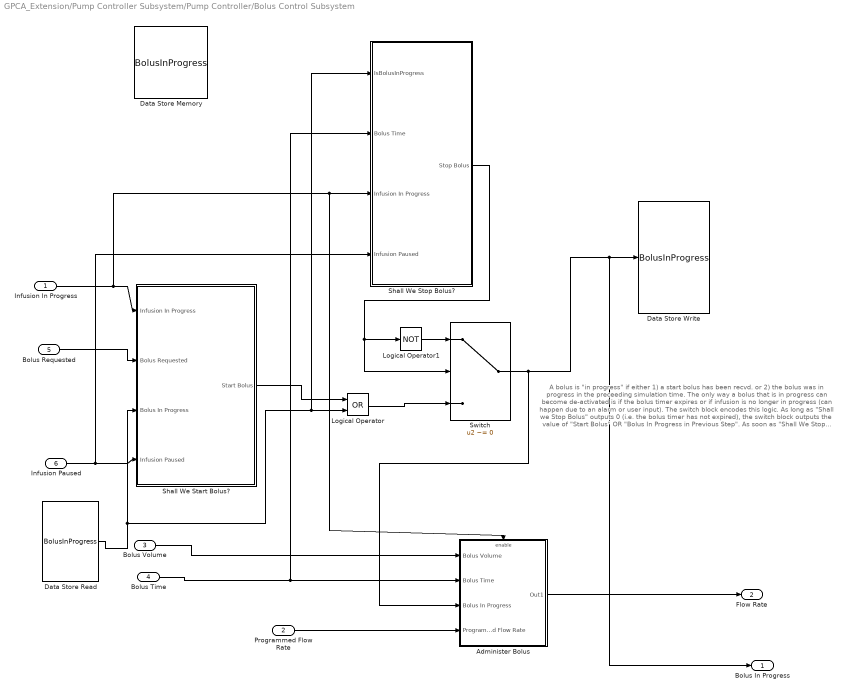
== system GPCA_Extension/Pump Controller Subsystem/Pump Controller/Bolus Control Subsystem ==
  note: A bolus is "in progress" if either 1) a start bolus has been recvd. or 2) the bolus was in progress
      | in the preceeding simulation time. The only way a bolus that is in progress can become de-activated is if the bolus
      | timer expires or if infusion is no longer in progress (can happen due to an alarm or user input).  The switch block encodes this logic.
      | As long as "Shall we Stop Bolus" outputs 0 (i.e. the bolus timer has not expired),
      | the switch block outputs the value of "Start Bolus" OR "Bolus In Progress in Previous Step".
      | As soon as "Shall We Stop Bolus" outputs 1,
      | the switch outputs 0.
  Infusion In Progress : Inport
  Programmed Flow Rate : Inport  Port=2
  Bolus Volume : Inport  Port=3
  Bolus Time : Inport  Port=4
  Bolus Requested : Inport  Port=5
  Infusion Paused : Inport  Port=6
  Administer Bolus : Subsystem
  Data Store Memory : DataStoreMemory  DataStoreName=BolusInProgress  OutDataTypeStr=boolean
  Data Store Read : DataStoreRead  DataStoreName=BolusInProgress
  Data Store Write : DataStoreWrite  DataStoreName=BolusInProgress
  Logical Operator : Logic  Operator=OR  AllPortsSameDT=off  OutDataTypeStr=boolean
  Logical Operator1 : Logic  Operator=NOT  AllPortsSameDT=off  OutDataTypeStr=boolean
  Shall We Start Bolus? : Subsystem
  Shall We Stop Bolus? : Subsystem
  Switch : Switch  Criteria=u2 ~= 0
  " Bolus In Progress" : Outport
  Flow Rate : Outport  Port=2
  wires:
  Infusion In Progress/1 -> Shall We Start Bolus?/1(Infusion In Progress), Shall We Stop Bolus?/3(Infusion In Progress), Administer Bolus/Enable
  Bolus Requested/1 -> Shall We Start Bolus?/2(Bolus Requested)
  Data Store Read/1 -> Shall We Start Bolus?/3(Bolus In Progress), Logical Operator/2, Shall We Stop Bolus?/1(IsBolusInProgress)
  Bolus Volume/1 -> Administer Bolus/1(Bolus Volume)
  Bolus Time/1 -> Administer Bolus/2(Bolus Time), Shall We Stop Bolus?/2(Bolus Time)
  Programmed Flow Rate/1 -> Administer Bolus/4(Programmed Flow Rate)
  Administer Bolus/1(Out1) -> Flow Rate/1
  Switch/1 -> Administer Bolus/3(Bolus In Progress), Data Store Write/1, " Bolus In Progress"/1
  Shall We Start Bolus?/1(Start Bolus) -> Logical Operator/1
  Shall We Stop Bolus?/1(Stop Bolus) -> Switch/2, Logical Operator1/1
  Logical Operator1/1 -> Switch/1
  Infusion Paused/1 -> Shall We Start Bolus?/4(Infusion Paused), Shall We Stop Bolus?/4(Infusion Paused)
  Logical Operator/1 -> Switch/3

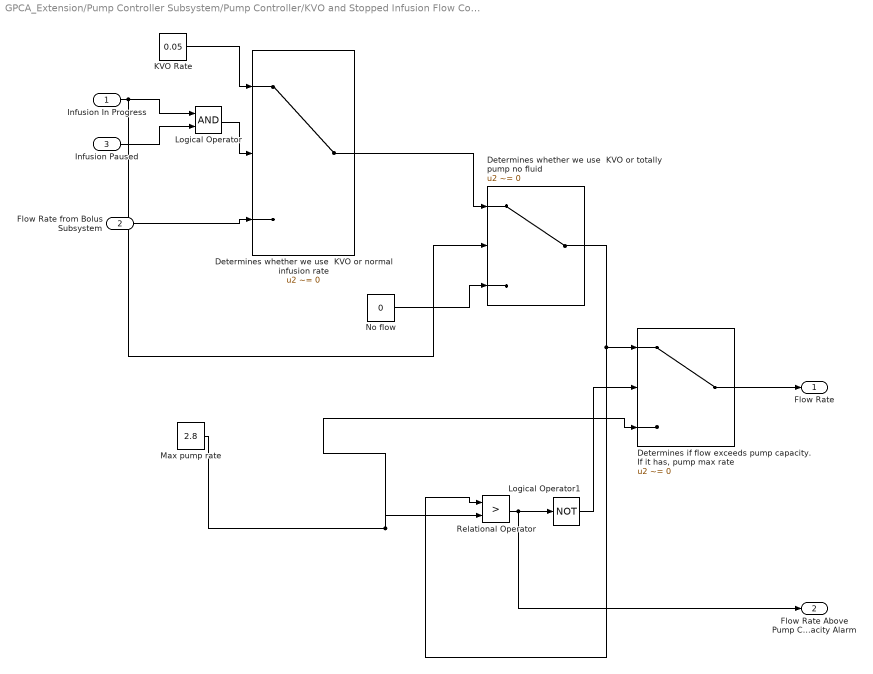
== system GPCA_Extension/Pump Controller Subsystem/Pump Controller/KVO and Stopped Infusion Flow Control Subsystem ==
  Infusion In Progress : Inport
  Flow Rate from Bolus Subsystem : Inport  Port=2
  Infusion Paused : Inport  Port=3
  "Determines if flow exceeds pump capacity. If it has, pump max rate" : Switch  Criteria=u2 ~= 0
  Determines whether we use  KVO or normal infusion rate : Switch  Criteria=u2 ~= 0
  Determines whether we use  KVO or totally pump no fluid : Switch  Criteria=u2 ~= 0
  KVO Rate : Constant  Value=0.05
  Logical Operator : Logic  AllPortsSameDT=off  OutDataTypeStr=boolean
  Logical Operator1 : Logic  Operator=NOT  AllPortsSameDT=off  OutDataTypeStr=boolean
  Max pump rate : Constant  Value=2.8
  No flow : Constant  Value=0
  Relational Operator : RelationalOperator  Operator=>  OutDataTypeStr=boolean
  Flow Rate : Outport
  " Flow Rate Above Pump Capacity Alarm" : Outport  Port=2
  wires:
  KVO Rate/1 -> Determines whether we use  KVO or normal infusion rate/1
  Flow Rate from Bolus Subsystem/1 -> Determines whether we use  KVO or normal infusion rate/3
  Infusion In Progress/1 -> Logical Operator/1, Determines whether we use  KVO or totally pump no fluid/2
  Infusion Paused/1 -> Logical Operator/2
  Logical Operator/1 -> Determines whether we use  KVO or normal infusion rate/2
  Determines whether we use  KVO or normal infusion rate/1 -> Determines whether we use  KVO or totally pump no fluid/1
  No flow/1 -> Determines whether we use  KVO or totally pump no fluid/3
  "Determines if flow exceeds pump capacity. If it has, pump max rate"/1 -> Flow Rate/1
  Determines whether we use  KVO or totally pump no fluid/1 -> "Determines if flow exceeds pump capacity. If it has, pump max rate"/1, Relational Operator/1
  Max pump rate/1 -> "Determines if flow exceeds pump capacity. If it has, pump max rate"/3, Relational Operator/2
  Relational Operator/1 -> Logical Operator1/1, " Flow Rate Above Pump Capacity Alarm"/1
  Logical Operator1/1 -> "Determines if flow exceeds pump capacity. If it has, pump max rate"/2

== system GPCA_Extension/Pump Controller Subsystem/Pump Controller/Bolus Control Subsystem/Administer Bolus ==
  Bolus Volume : Inport
  Bolus Time : Inport  Port=2
  Bolus In Progress : Inport  Port=3
  Programmed Flow Rate : Inport  Port=4
  Enable : EnablePort
  Divide : Product  Inputs=*/
  Switch : Switch  Criteria=u2 ~= 0
  Out1 : Outport
  wires:
  Bolus Volume/1 -> Divide/1
  Bolus Time/1 -> Divide/2
  Divide/1 -> Switch/1
  Bolus In Progress/1 -> Switch/2
  Switch/1 -> Out1/1
  Programmed Flow Rate/1 -> Switch/3

== system GPCA_Extension/Pump Controller Subsystem/Pump Controller/Bolus Control Subsystem/Shall We Start Bolus? ==
  Infusion In Progress : Inport
  Bolus Requested : Inport  Port=2
  Bolus In Progress : Inport  Port=3
  Infusion Paused : Inport  Port=4
  Logical Operator1 : Logic  Operator=NOT  AllPortsSameDT=off  OutDataTypeStr=boolean
  Logical Operator2 : Logic  Inputs=4  OutDataTypeStr=boolean
  Logical Operator3 : Logic  Operator=NOT  AllPortsSameDT=off  OutDataTypeStr=boolean
  Start Bolus : Outport
  wires:
  Bolus Requested/1 -> Logical Operator2/2
  Bolus In Progress/1 -> Logical Operator1/1
  Infusion In Progress/1 -> Logical Operator2/1
  Logical Operator1/1 -> Logical Operator2/3
  Logical Operator2/1 -> Start Bolus/1
  Logical Operator3/1 -> Logical Operator2/4
  Infusion Paused/1 -> Logical Operator3/1

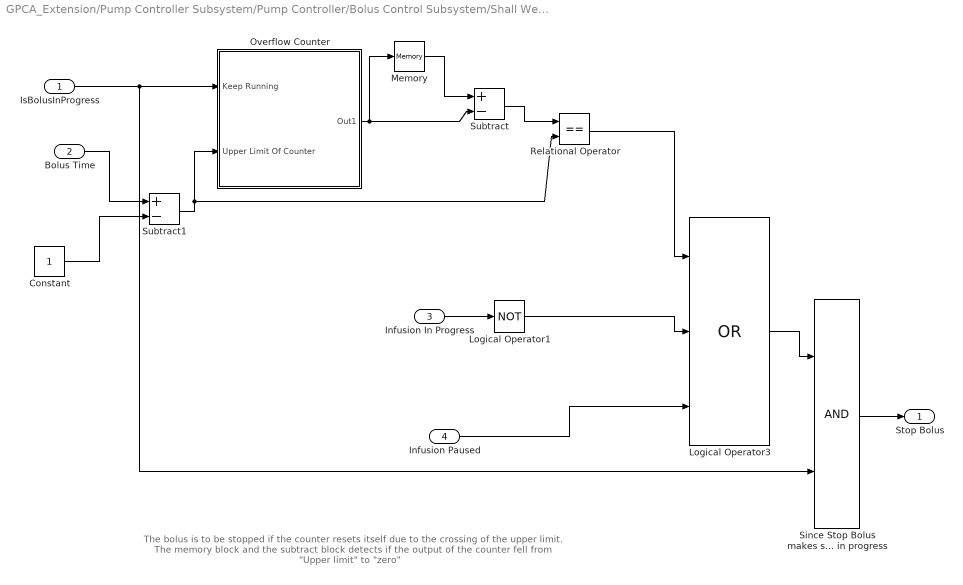
== system GPCA_Extension/Pump Controller Subsystem/Pump Controller/Bolus Control Subsystem/Shall We Stop Bolus? ==
  note: The bolus is to be stopped if the counter resets itself due to
      | the crossing of the upper limit. The memory block and the subtract block
      | detects if the output of the counter fell from "Upper limit" to "zero"
  IsBolusInProgress : Inport
  Bolus Time : Inport  Port=2
  Infusion In Progress : Inport  Port=3
  Infusion Paused : Inport  Port=4
  Constant : Constant
  Logical Operator1 : Logic  Operator=NOT  AllPortsSameDT=off  OutDataTypeStr=boolean
  Logical Operator3 : Logic  Operator=OR  Inputs=3  AllPortsSameDT=off  OutDataTypeStr=boolean
  Memory : Memory  InheritSampleTime=on
  Overflow Counter : Subsystem
  Relational Operator : RelationalOperator  Operator===  OutDataTypeStr=boolean
  Since Stop Bolus makes sense only when there was bolus in progress : Logic  AllPortsSameDT=off  OutDataTypeStr=boolean
  Subtract : Sum  Inputs=+-
  Subtract1 : Sum  Inputs=+-
  Stop Bolus : Outport
  wires:
  Overflow Counter/1(Out1) -> Memory/1, Subtract/2
  IsBolusInProgress/1 -> Overflow Counter/1(Keep Running), Since Stop Bolus makes sense only when there was bolus in progress/2
  Memory/1 -> Subtract/1
  Subtract/1 -> Relational Operator/1
  Relational Operator/1 -> Logical Operator3/1
  Infusion In Progress/1 -> Logical Operator1/1
  Logical Operator1/1 -> Logical Operator3/2
  Infusion Paused/1 -> Logical Operator3/3
  Since Stop Bolus makes sense only when there was bolus in progress/1 -> Stop Bolus/1
  Logical Operator3/1 -> Since Stop Bolus makes sense only when there was bolus in progress/1
  Bolus Time/1 -> Subtract1/1
  Constant/1 -> Subtract1/2
  Subtract1/1 -> Overflow Counter/2(Upper Limit Of Counter), Relational Operator/2

== system GPCA_Extension/Pump Controller Subsystem/Pump Controller/Bolus Control Subsystem/Shall We Stop Bolus?/Overflow Counter ==
  Keep Running : Inport
  Upper Limit Of Counter : Inport  Port=2
  Add : Sum
  Constant : Constant  Value=0
  Constant1 : Constant
  Counter : UnitDelay
  Logical Operator : Logic  AllPortsSameDT=off  OutDataTypeStr=boolean
  Update counter : Switch  Threshold=1
  Value of Counter Less Than Threshold : RelationalOperator  Operator=<  OutDataTypeStr=boolean
  Out1 : Outport
  wires:
  Add/1 -> Update counter/1
  Constant1/1 -> Add/1
  Counter/1 -> Add/2, Value of Counter Less Than Threshold/1
  Update counter/1 -> Counter/1, Out1/1
  Upper Limit Of Counter/1 -> Value of Counter Less Than Threshold/2
  Constant/1 -> Update counter/3
  Keep Running/1 -> Logical Operator/1
  Value of Counter Less Than Threshold/1 -> Logical Operator/2
  Logical Operator/1 -> Update counter/2
